simulink model "main_to_linearize"  (R2025b)
settings: Solver=FixedStepAuto  StartTime=0  StopTime=100  FixedStep=sample_time  RelTol=1e-3
undefined symbols (not defined in the file or in its folder): A_cut_in, control_allocator_matrix, f_xy_tf, fractalcoef, G_rate, initial_euler, K_coeff, mav_inertia_ctrl, mav_mass, phase_lag, thrust_coeff_bot, thrust_coeff_top, thrust_tf, top_motor_arm, torque_coeff_bot, torque_coeff_top
libraries: aerolibobsolete x1, matrix_library x1, aerolibutil x1, uavutilslib x1, sensorgpslib x1, mspsensorlib x1, sharedtransform x1
settings Model: Creator=tommy  LastModifiedBy=tommy
settings DataIOCC: SaveFormat=StructureWithTime
settings OptimizationCC: BlockReduction=off  DefaultParameterBehavior=Inlined  UseDivisionForNetSlopeComputation=on  GainParamInheritBuiltInType=on  UseFloatMulNetSlope=on  InlineInvariantSignals=on  OptimizeBlockIOStorage=off  BufferReuse=off  EnhancedBackFolding=on  BooleansAsBitfields=on  PassReuseOutputArgsAs=Individual arguments  StateBitsets=on  DataBitsets=on  ZeroExternalMemoryAtStartup=off  ZeroInternalMemoryAtStartup=off  NoFixptDivByZeroProtection=on  EfficientFloat2IntCast=on  LifeSpan=1  OptimizeBlockOrder=speed  DifferentSizesBufferReuse=on  EfficientTunableParamExpr=on
settings DebuggingCC: AlgebraicLoopMsg=none  ParameterTunabilityLossMsg=error
settings HardwareCC: ProdBitPerPointer=32.0  ProdBitPerSizeT=32.0  ProdBitPerPtrDiffT=32.0  ProdLargestAtomicInteger=Long  ProdLargestAtomicFloat=Double  ProdWordSize=32.0  ProdLongLongMode=on  ProdHWDeviceType=ARM Compatible->ARM Cortex-M
settings SFSimCC: MATLABDynamicMemAlloc=off  SimTargetLang=C++  SimDLTargetLibrary=mkl-dnn
settings RTWCC: SystemTargetFile=ert.tlc  TemplateMakefile=ert_default_tmf  TargetLang=C++  Description=Embedded Coder
settings CodeAppCC: ForceParamTrailComments=on  IgnoreCustomStorageClasses=off  OperatorAnnotations=on  SimulinkDataObjDesc=on  SFDataObjDesc=on  CustomSymbolStrGlobalVar=rt$N$M  CustomSymbolStrType=$N$M  CustomSymbolStrFcn=$N$M$F  CustomSymbolStrMacro=$N$M  InsertBlockDesc=on
settings ERTTargetCC: RootIOFormat=Structure reference  ERTCustomFileTemplate=example_file_process.tlc  ERTFilePackagingFormat=CompactWithDataFile  TargetLangStandard=C++11 (ISO)  GenerateSampleERTMain=on  IncludeMdlTerminateFcn=off  CombineSignalStateStructs=on  SuppressErrorStatus=on  SupportAbsoluteTime=off  CodeInterfacePackaging=C++ class  SupportComplex=off

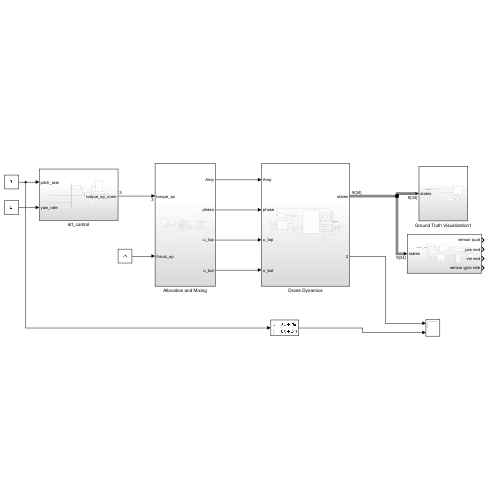
[thumbnail: Simulink's stored preview of the top-level diagram]
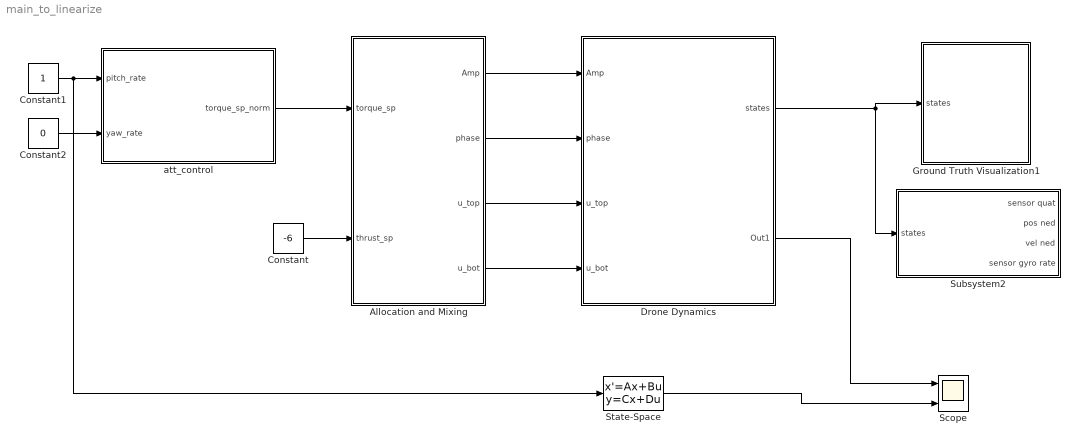
== system main_to_linearize ==
  Allocation and Mixing : Subsystem
  Constant : Constant  Value=-6
  Constant1 : Constant
  Constant2 : Constant  Value=0
  Drone Dynamics : Subsystem
  Ground Truth Visualization1 : Subsystem
  Scope : Scope  NumInputPorts=2
      settings: ActiveDisplayYMinimum=-0.027502183386848192  ActiveDisplayYMaximum=0.021746809856548664  DataLoggingVariableName=ScopeData2
  State-Space : StateSpace  A=G_rate.A  B=G_rate.B  C=G_rate.C  D=G_rate.D  InitialCondition=0
  Subsystem2 : Subsystem
  att_control : Subsystem
  wires:
  Drone Dynamics/1(states) -> Subsystem2/1(states), Ground Truth Visualization1/1(states)
  Allocation and Mixing/2(phase) -> Drone Dynamics/2(phase)
  Allocation and Mixing/3(u_top) -> Drone Dynamics/3(u_top)
  Allocation and Mixing/4(u_bot) -> Drone Dynamics/4(u_bot)
  Allocation and Mixing/1(Amp) -> Drone Dynamics/1(Amp)
  Constant/1 -> Allocation and Mixing/2(thrust_sp)
  att_control/1(torque_sp_norm) -> Allocation and Mixing/1(torque_sp)
  Constant2/1 -> att_control/2(yaw_rate)
  Drone Dynamics/2(Out1) -> Scope/1
  State-Space/1 -> Scope/2
  Constant1/1 -> State-Space/1, att_control/1(pitch_rate)

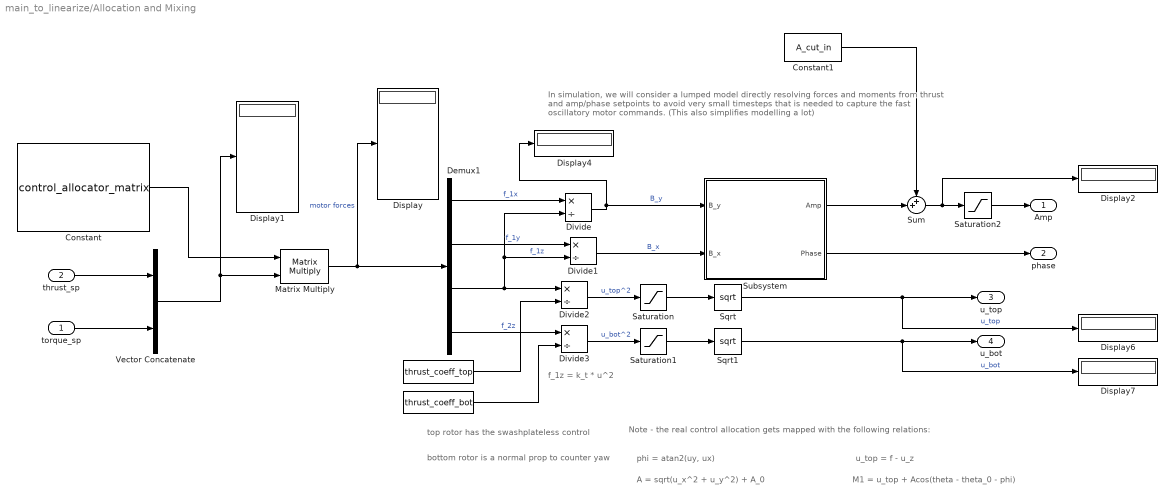
== system main_to_linearize/Allocation and Mixing ==
  note: f_1z = k_t * u^2
  note: u_top = f - u_z
  note: In simulation, we will consider a lumped model directly resolving forces and moments from thrust and amp/phase setpoints to avoid very small timesteps that is needed to capture the fast oscillatory motor commands. (This also simplifies modelling a lot)
  note: phi = atan2(uy, ux)
  note: A = sqrt(u_x^2 + u_y^2) + A_0
  note: top rotor has the swashplateless control
  note: bottom rotor is a normal prop to counter yaw
  note: Note - the real control allocation gets mapped with the following relations:
  note: M1 = u_top + Acos(theta - theta_0 - phi)
  torque_sp : Inport
  thrust_sp : Inport  Port=2
  " " : Constant  Value=thrust_coeff_top
  "  " : Constant  Value=thrust_coeff_bot
  Constant : Constant  Value=control_allocator_matrix
  Constant1 : Constant  Value=A_cut_in
  Demux1 : Demux
  Display{,1..2,4,6..7} (6 alike) : Display
  Divide{,1..3} (4 alike) : Product  Inputs=*/
  Matrix Multiply : Product  Multiplication=Matrix(*)
  Saturation : Saturate  UpperLimit=1  LowerLimit=0
  Saturation1 : Saturate  UpperLimit=1  LowerLimit=0
  Saturation2 : Saturate  UpperLimit=0.3  LowerLimit=0
  Sqrt : Sqrt
  Sqrt1 : Sqrt
  Subsystem : Subsystem
  Sum : Sum  Inputs=++|
  Vector Concatenate : Concatenate
  Amp : Outport
  phase : Outport  Port=2
  u_top : Outport  Port=3
  u_bot : Outport  Port=4
  wires:
  Divide/1 -> Subsystem/1(B_y), Display4/1  "B_y"
  Demux1/2 -> Divide1/1  "f_1y"
  Sqrt/1 -> u_top/1, Display6/1  "u_top"
  Sqrt1/1 -> u_bot/1, Display7/1  "u_bot"
  torque_sp/1 -> Vector Concatenate/2
  Constant/1 -> Matrix Multiply/1
  thrust_sp/1 -> Vector Concatenate/1
  Vector Concatenate/1 -> Display1/1, Matrix Multiply/2
  Matrix Multiply/1 -> Display/1, Demux1/1  "motor forces"
  Sum/1 -> Display2/1, Saturation2/1
  Constant1/1 -> Sum/1
  Saturation2/1 -> Amp/1
  Demux1/1 -> Divide/1  "f_1x"
  Demux1/3 -> Divide/2, Divide1/2, Divide2/1  "f_1z"
  Demux1/4 -> Divide3/1  "f_2z"
  " "/1 -> Divide2/2
  "  "/1 -> Divide3/2
  Divide2/1 -> Saturation/1  "u_top^2"
  Divide3/1 -> Saturation1/1  "u_bot^2"
  Saturation/1 -> Sqrt/1
  Saturation1/1 -> Sqrt1/1
  Divide1/1 -> Subsystem/2(B_x)  "B_x"
  Subsystem/2(Phase) -> phase/1
  Subsystem/1(Amp) -> Sum/2

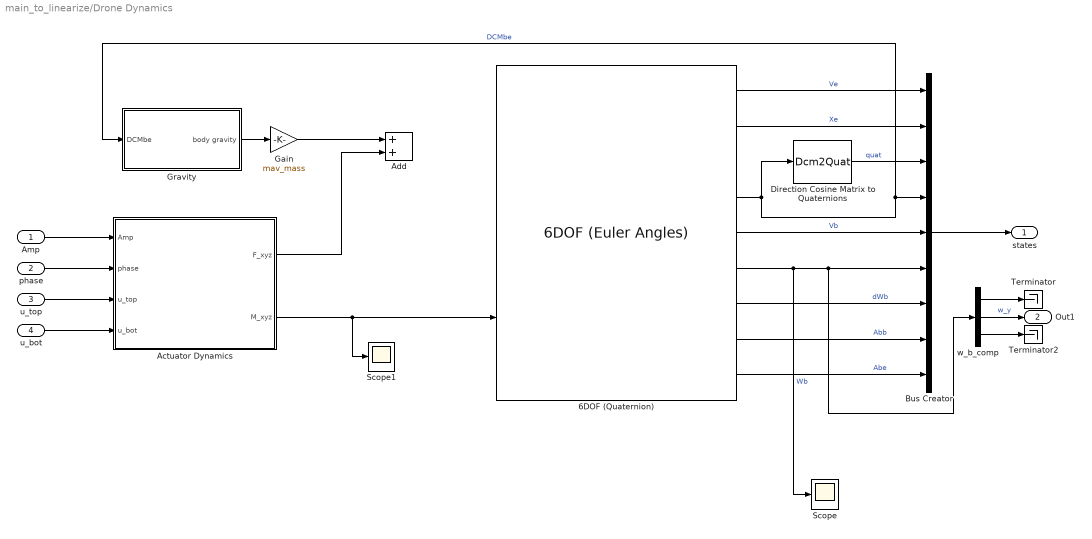
== system main_to_linearize/Drone Dynamics ==
  Amp : Inport
  phase : Inport  Port=2
  u_top : Inport  Port=3
  u_bot : Inport  Port=4
  6DOF (Quaternion) : aerolibobsolete/6DOF (Euler Angles)  units=Metric (MKS)  mtype=Fixed  rep=Quaternion  xme_0=[0 0 0]  Vm_0=[0 0 0]  eul_0=initial_euler  pm_0=[0 0 0]  mass_0=mav_mass  mass_e=0.5  mass_f=2.0  inertia=mav_inertia  inertia_e=eye(3)  inertia_f=2*eye(3)  k_quat=1.0  vre_flag=on  abi_flag=on  aMode=0  xme_statename=''  Vm_statename=''  eul_statename=''  quat_statename=''  pm_statename=''  mass_statename=''
  Actuator Dynamics : Subsystem
  Add : Sum
  Bus Creator : BusCreator  Inputs=9
  Direction Cosine Matrix to Quaternions : Dcm2Quat
  Gain : Gain  Gain=mav_mass
  Gravity : Subsystem
  Scope : Scope
      settings: ActiveDisplayYMinimum=-3.1765505415243829  ActiveDisplayYMaximum=3.0646959132907146  DataLoggingVariableName=ScopeData8
  Scope1 : Scope
      settings: ActiveDisplayYMinimum=-0.093468111798381326  ActiveDisplayYMaximum=0.1127572791811684  DataLoggingVariableName=ScopeData5
  Terminator : Terminator
  Terminator2 : Terminator
  w_b_comp : Demux  Outputs=3
  states : Outport
  Out1 : Outport  Port=2
  wires:
  6DOF (Quaternion)/7 -> Bus Creator/7  "dWb"
  6DOF (Quaternion)/8 -> Bus Creator/8  "Abb"
  6DOF (Quaternion)/6 -> Scope/1, w_b_comp/1, Bus Creator/6  "Wb"
  u_bot/1 -> Actuator Dynamics/4(u_bot)
  Bus Creator/1 -> states/1
  6DOF (Quaternion)/9 -> Bus Creator/9  "Abe"
  phase/1 -> Actuator Dynamics/2(phase)
  6DOF (Quaternion)/1 -> Bus Creator/1  "Ve"
  6DOF (Quaternion)/2 -> Bus Creator/2  "Xe"
  Amp/1 -> Actuator Dynamics/1(Amp)
  6DOF (Quaternion)/5 -> Bus Creator/5  "Vb"
  6DOF (Quaternion)/4 -> Bus Creator/4, Gravity/1(DCMbe), Direction Cosine Matrix to Quaternions/1  "DCMbe"
  Actuator Dynamics/1(F_xyz) -> Add/2
  Gravity/1(body gravity) -> Gain/1
  Gain/1 -> Add/1
  Actuator Dynamics/2(M_xyz) -> Scope1/1, 6DOF (Quaternion)/2
  Direction Cosine Matrix to Quaternions/1 -> Bus Creator/3  "quat"
  u_top/1 -> Actuator Dynamics/3(u_top)
  w_b_comp/1 -> Terminator/1
  w_b_comp/3 -> Terminator2/1
  w_b_comp/2 -> Out1/1  "w_y"

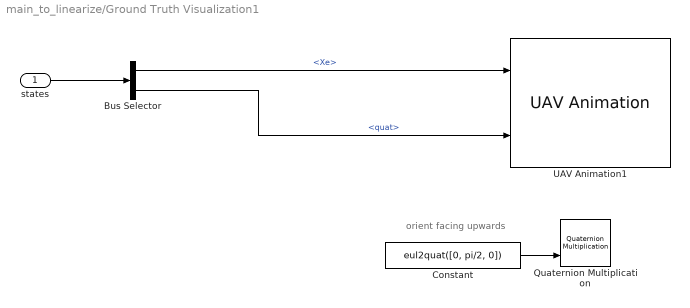
== system main_to_linearize/Ground Truth Visualization1 ==
  note: orient facing upwards
  states : Inport
  Bus Selector : BusSelector  OutputSignals=Xe,quat
  Constant : Constant  Value=eul2quat([0, pi/2, 0])  VectorParams1D=off
  Quaternion Multiplication : aerolibutil/Quaternion Multiplication
  UAV Animation1 : uavutilslib/UAV Animation  NumUAV=1  DynamicUAVConfig=off  UAVType=Multirotor  UAVSize=1  UAVColor=[1 0 0]  UAVTrajectoryAlpha=1  InertialZDirection=Down  RotationFormat=Quaternion  DrawMarkers=off  SampleTime=0.05
  wires:
  states/1 -> Bus Selector/1
  Bus Selector/1 -> UAV Animation1/1  "<Xe>"
  Bus Selector/2 -> UAV Animation1/2  "<quat>"
  Constant/1 -> Quaternion Multiplication/2

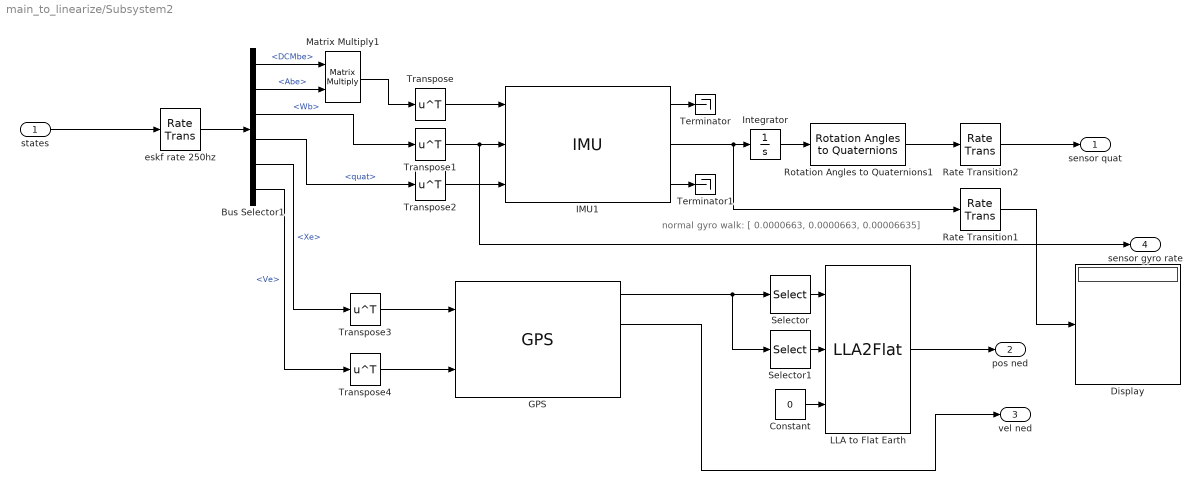
== system main_to_linearize/Subsystem2 ==
  note: normal gyro walk: [ 0.0000663, 0.0000663, 0.00006635]
  states : Inport
  Bus Selector1 : BusSelector  OutputSignals=DCMbe,Abe,Wb,quat,Xe,Ve
  Constant : Constant  Value=0
  Display : Display
  GPS : sensorgpslib/GPS  DispRefFrame=NED  PositionInputFormat=Local  ReferenceLocation=[ 43.660624994362166, -79.39579849130422, 0 ]  HorizontalPositionAccuracy=1.6  VerticalPositionAccuracy=2  VelocityAccuracy=0.1  DecayFactor=0.999  SeedDouble=67  SimulateUsing=Interpreted execution
      settings: LibrarySourceBlock=uavsimlib/GPS
  IMU1 : mspsensorlib/IMU  DispRefFrame=NED  TemperaturePort=off  Temperature=0  MagneticFieldPort=off  MagneticFieldNED=[ 27.5550, -2.4169, -16.0849 ]  MagneticFieldENU=[ -2.4169, 27.5550, 16.0849 ]  SeedDouble=67  SimulateUsing=Interpreted execution  AccelParamsMeasurementRange=Inf  AccelParamsResolution=0  AccelParamsConstantBias=[ 0, 0, 0 ]  AccelParamsAxesMisalignment=[ 1, 0, 0; 0, 1, 0; 0, 0, 1 ]  AccelParamsNoiseDensity=[ 0, 0, 0 ]  AccelParamsBiasInstability=[ 0, 0, 0 ]  AccelParamsBiasInstabilityNumerator=fractalcoef().Numerator  AccelParamsBiasInstabilityDenominator=fractalcoef().Denominator  AccelParamsRandomWalk=[ 0, 0, 0 ]  AccelParamsNoiseType=double-sided  AccelParamsTemperatureBias=[ 0, 0, 0 ]  AccelParamsTemperatureScaleFactor=[ 0, 0, 0 ]  GyroParamsMeasurementRange=Inf  GyroParamsResolution=0  GyroParamsConstantBias=[ 0, 0, 0 ]  GyroParamsAxesMisalignment=[ 100, 0, 0; 0, 100, 0; 0, 0, 100 ]  GyroParamsAccelerationBias=[ 0, 0, 0 ]  GyroParamsNoiseDensity=[0, 0, 0]  GyroParamsBiasInstability=[ 0, 0, 0 ]  GyroParamsBiasInstabilityNumerator=fractalcoef().Numerator  GyroParamsBiasInstabilityDenominator=fractalcoef().Denominator  GyroParamsRandomWalk=[ 0, 0, 0 ]  GyroParamsNoiseType=double-sided  GyroParamsTemperatureBias=[ 0, 0, 0 ]  GyroParamsTemperatureScaleFactor=[ 0, 0, 0 ]  MagParamsMeasurementRange=Inf  MagParamsResolution=0  MagParamsConstantBias=[ 0, 0, 0 ]  MagParamsAxesMisalignment=[ 100, 0, 0; 0, 100, 0; 0, 0, 100 ]  MagParamsNoiseDensity=[ 0, 0, 0 ]  MagParamsBiasInstability=[ 0, 0, 0 ]  MagParamsBiasInstabilityNumerator=fractalcoef().Numerator  MagParamsBiasInstabilityDenominator=fractalcoef().Denominator  MagParamsRandomWalk=[ 0, 0, 0 ]  MagParamsNoiseType=double-sided  MagParamsTemperatureBias=[ 0, 0, 0 ]  MagParamsTemperatureScaleFactor=[ 0, 0, 0 ]
  Integrator : Integrator  InitialCondition=initial_euler
  LLA to Flat Earth : LLA2Flat  LL0=[43.660624994362166, -79.39579849130422]
  Matrix Multiply1 : Product  Multiplication=Matrix(*)
  Rate Transition1 : RateTransition  OutPortSampleTime=1/1000
  Rate Transition2 : RateTransition  OutPortSampleTime=1/250
  Rotation Angles to Quaternions1 : sharedtransform/Rotation Angles to Quaternions  rotationOrder=XYZ  aMode=aMode
  Selector : Selector  InputPortWidth=3  IndexOptions=Index vector (dialog)  Indices=[1 2]  OutputSizes=1
  Selector1 : Selector  InputPortWidth=3  IndexOptions=Index vector (dialog)  Indices=[3]  OutputSizes=1
  Terminator : Terminator
  Terminator1 : Terminator
  Transpose{,1..4} (5 alike) : Math  Operator=transpose
  eskf rate 250hz : RateTransition  OutPortSampleTime=1/250
  sensor quat : Outport
  pos ned : Outport  Port=2
  vel ned : Outport  Port=3
  sensor gyro rate : Outport  Port=4
  wires:
  Transpose1/1 -> IMU1/2, sensor gyro rate/1
  IMU1/2 -> Integrator/1, Rate Transition1/1
  Matrix Multiply1/1 -> Transpose/1
  Transpose/1 -> IMU1/1
  Integrator/1 -> Rotation Angles to Quaternions1/1
  Transpose2/1 -> IMU1/3
  Bus Selector1/4 -> Transpose2/1  "<quat>"
  Bus Selector1/3 -> Transpose1/1  "<Wb>"
  Rotation Angles to Quaternions1/1 -> Rate Transition2/1
  states/1 -> eskf rate 250hz/1
  eskf rate 250hz/1 -> Bus Selector1/1
  IMU1/1 -> Terminator/1
  IMU1/3 -> Terminator1/1
  Bus Selector1/1 -> Matrix Multiply1/1  "<DCMbe>"
  Bus Selector1/2 -> Matrix Multiply1/2  "<Abe>"
  Rate Transition1/1 -> Display/1
  Rate Transition2/1 -> sensor quat/1
  GPS/1 -> Selector1/1, Selector/1
  Selector/1 -> LLA to Flat Earth/1
  Selector1/1 -> LLA to Flat Earth/2
  Constant/1 -> LLA to Flat Earth/3
  GPS/2 -> vel ned/1
  LLA to Flat Earth/1 -> pos ned/1
  Bus Selector1/6 -> Transpose4/1  "<Ve>"
  Bus Selector1/5 -> Transpose3/1  "<Xe>"
  Transpose3/1 -> GPS/1
  Transpose4/1 -> GPS/2

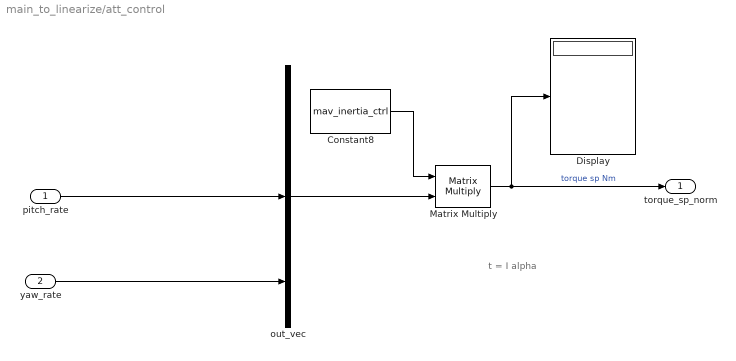
== system main_to_linearize/att_control ==
  note: t = I alpha
  pitch_rate : Inport
  yaw_rate : Inport  Port=2
  Constant8 : Constant  Value=mav_inertia_ctrl
  Display : Display
  Matrix Multiply : Product  Multiplication=Matrix(*)
  out_vec : Concatenate  NumInputs=3
  torque_sp_norm : Outport
  wires:
  Matrix Multiply/1 -> Display/1, torque_sp_norm/1  "torque sp Nm"
  Constant8/1 -> Matrix Multiply/1
  out_vec/1 -> Matrix Multiply/2
  pitch_rate/1 -> out_vec/2
  yaw_rate/1 -> out_vec/3

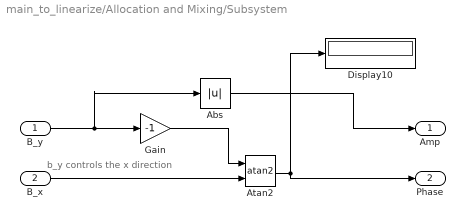
== system main_to_linearize/Allocation and Mixing/Subsystem ==
  note: b_y controls the x direction
  B_y : Inport
  B_x : Inport  Port=2
  Abs : Abs  SaturateOnIntegerOverflow=off
  Atan2 : Trigonometry  Operator=atan2
  Display10 : Display
  Gain : Gain  Gain=-1
  Amp : Outport
  Phase : Outport  Port=2
  wires:
  B_x/1 -> Atan2/2
  B_y/1 -> Abs/1, Gain/1
  Atan2/1 -> Phase/1, Display10/1
  Gain/1 -> Atan2/1
  Abs/1 -> Amp/1

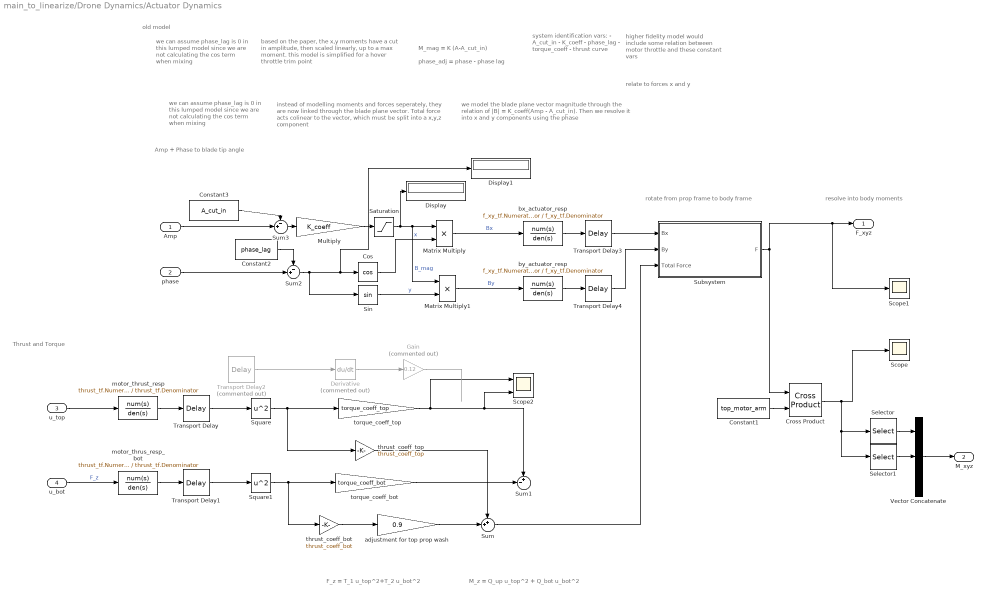
== system main_to_linearize/Drone Dynamics/Actuator Dynamics ==
  note: Amp + Phase to blade tip angle
  note: Thrust and Torque
  note: old model
  note: relate to forces x and y
  note: we can assume phase_lag is 0 in this lumped model since we are not calculating the cos term when mixing
  note: higher fidelity model would include some relation between motor throttle and these constant vars
  note: system identification vars:
      | - A_cut_in
      | - K_coeff
      | - phase_lag
      | - torque_coeff
      | - thrust curve
  note: M_mag = K (A-A_cut_in)
  note: based on the paper, the x,y moments have a cut in amplitude, then scaled linearly, up to a max moment. this model is simplified for a hover throttle trim point
  note: phase_adj = phase - phase lag
  note: M_z = Q_up u_top^2 + Q_bot u_bot^2
  note: F_z = T_1 u_top^2+T_2 u_bot^2
  note: resolve into body moments
  note: we can assume phase_lag is 0 in this lumped model since we are not calculating the cos term when mixing
  note: instead of modelling moments and forces seperately, they are now linked through the blade plane vector. Total force acts colinear to the vector, which must be split into a x,y,z component
  note: we model the blade plane vector magnitude through the relation of |B| = K_coeff(Amp - A_cut_in). Then we resolve it into x and y components using the phase
  note: rotate from prop frame to body frame
  Amp : Inport
  phase : Inport  Port=2
  u_top : Inport  Port=3
  u_bot : Inport  Port=4
  Constant1 : Constant  Value=top_motor_arm
  Constant2 : Constant  Value=phase_lag
  Constant3 : Constant  Value=A_cut_in
  Cos : Trigonometry  Operator=cos
  Cross Product : matrix_library/Cross Product
  Derivative : Derivative  Commented=on
  Display : Display
  Display1 : Display
  Gain : Gain  Commented=on  Gain=0.12
  Matrix Multiply : Product
  Matrix Multiply1 : Product
  Multiply : Gain  Gain=K_coeff
  Saturation : Saturate  UpperLimit=inf  LowerLimit=0
  Scope : Scope
      settings: ActiveDisplayYMinimum=-0.0046517365862840283  ActiveDisplayYMaximum=0.012758813227963812
  Scope1 : Scope
      settings: ActiveDisplayYMinimum=-1  ActiveDisplayYMaximum=1
  Scope2 : Scope  NumInputPorts=2
      settings: ActiveDisplayYMinimum=-0.016923057380667912  ActiveDisplayYMaximum=0.1375268910048818  DataLoggingVariableName=ScopeData10
  Selector : Selector  InputPortWidth=3  IndexOptions=Index vector (dialog)  Indices=[1]  OutputSizes=1
  Selector1 : Selector  InputPortWidth=3  IndexOptions=Index vector (dialog)  Indices=[2]  OutputSizes=1
  Sin : Trigonometry
  Square : Math  Operator=square
  Square1 : Math  Operator=square
  Subsystem : Subsystem
  Sum : Sum  Inputs=++|
  Sum1 : Sum  Inputs=+-|
  Sum2 : Sum  Inputs=-+|
  Sum3 : Sum  Inputs=-+|
  Transport Delay : TransportDelay  DelayTime=0.15  TransDelayFeedthrough=on  PadeOrder=1
  Transport Delay1 : TransportDelay  DelayTime=0.15  TransDelayFeedthrough=on  PadeOrder=1
  Transport Delay2 : TransportDelay  Commented=on  DelayTime=0.1
  Transport Delay3 : TransportDelay  DelayTime=0.1  TransDelayFeedthrough=on  PadeOrder=1
  Transport Delay4 : TransportDelay  DelayTime=0.1  TransDelayFeedthrough=on  PadeOrder=1
  Vector Concatenate : Concatenate  NumInputs=3
  adjustment for top prop wash : Gain  Gain=0.9
  bx_actuator_resp : TransferFcn  Numerator=f_xy_tf.Numerator  Denominator=f_xy_tf.Denominator
  by_actuator_resp : TransferFcn  Numerator=f_xy_tf.Numerator  Denominator=f_xy_tf.Denominator
  motor_thrus_resp_bot : TransferFcn  Numerator=thrust_tf.Numerator  Denominator=thrust_tf.Denominator
  motor_thrust_resp : TransferFcn  Numerator=thrust_tf.Numerator  Denominator=thrust_tf.Denominator
  thrust_coeff_bot : Gain  Gain=thrust_coeff_bot
  thrust_coeff_top : Gain  Gain=thrust_coeff_top
  torque_coeff_bot : Gain  Gain=torque_coeff_bot
  torque_coeff_top : Gain  Gain=torque_coeff_top
  F_xyz : Outport
  M_xyz : Outport  Port=2
  wires:
  u_bot/1 -> motor_thrus_resp_bot/1  "F_z"
  Constant2/1 -> Sum2/1
  phase/1 -> Sum2/2
  Sum2/1 -> Sin/1, Cos/1, Display1/1
  Amp/1 -> Sum3/2
  Constant3/1 -> Sum3/1
  Sum3/1 -> Multiply/1
  Multiply/1 -> Saturation/1
  Cos/1 -> Matrix Multiply/2  "x"
  Matrix Multiply1/1 -> by_actuator_resp/1  "By"
  Sin/1 -> Matrix Multiply1/2  "y"
  Saturation/1 -> Display/1, Matrix Multiply1/1, Matrix Multiply/1  "B_mag"
  Constant1/1 -> Cross Product/2
  Cross Product/1 -> Selector1/1, Selector/1, Scope/1
  Subsystem/1(F) -> Scope1/1, F_xyz/1, Cross Product/1
  by_actuator_resp/1 -> Transport Delay4/1
  bx_actuator_resp/1 -> Transport Delay3/1
  Square/1 -> torque_coeff_top/1, thrust_coeff_top/1
  Square1/1 -> thrust_coeff_bot/1, torque_coeff_bot/1
  Vector Concatenate/1 -> M_xyz/1
  Selector/1 -> Vector Concatenate/1
  Selector1/1 -> Vector Concatenate/2
  torque_coeff_bot/1 -> Sum1/2
  Matrix Multiply/1 -> bx_actuator_resp/1  "Bx"
  thrust_coeff_bot/1 -> adjustment for top prop wash/1
  torque_coeff_top/1 -> Scope2/2, Sum1/1, Scope2/1
  u_top/1 -> motor_thrust_resp/1
  thrust_coeff_top/1 -> Sum/1
  adjustment for top prop wash/1 -> Sum/2
  Derivative/1 -> Gain/1
  Gain/1 -> ?
  Transport Delay2/1 -> Derivative/1
  Sum/1 -> Subsystem/3(Total Force)
  ? -> Transport Delay2/1
  motor_thrus_resp_bot/1 -> Transport Delay1/1
  motor_thrust_resp/1 -> Transport Delay/1
  Transport Delay/1 -> Square/1
  Transport Delay1/1 -> Square1/1
  Transport Delay3/1 -> Subsystem/1(Bx)
  Transport Delay4/1 -> Subsystem/2(By)

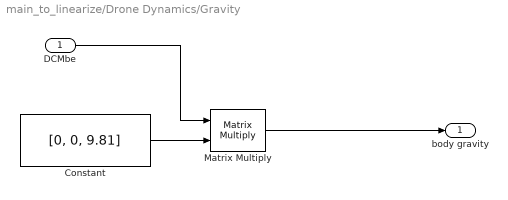
== system main_to_linearize/Drone Dynamics/Gravity ==
  DCMbe : Inport
  Constant : Constant  Value=[0, 0, 9.81]
  Matrix Multiply : Product  Multiplication=Matrix(*)
  body gravity : Outport
  wires:
  DCMbe/1 -> Matrix Multiply/1
  Constant/1 -> Matrix Multiply/2
  Matrix Multiply/1 -> body gravity/1

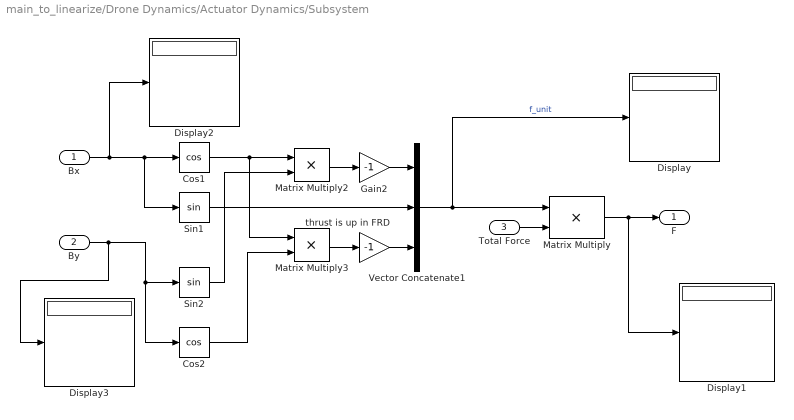
== system main_to_linearize/Drone Dynamics/Actuator Dynamics/Subsystem ==
  Bx : Inport
  By : Inport  Port=2
  Total Force : Inport  Port=3
  Cos1 : Trigonometry  Operator=cos
  Cos2 : Trigonometry  Operator=cos
  Display{,1..3} (4 alike) : Display
  Gain2 : Gain  Gain=-1
  Matrix Multiply : Product
  Matrix Multiply2 : Product
  Matrix Multiply3 : Product
  Sin1 : Trigonometry
  Sin2 : Trigonometry
  Vector Concatenate1 : Concatenate  NumInputs=3
  thrust is up in FRD : Gain  Gain=-1
  F : Outport
  wires:
  Sin1/1 -> Vector Concatenate1/2
  Bx/1 -> Display2/1, Sin1/1, Cos1/1
  Cos1/1 -> Matrix Multiply3/1, Matrix Multiply2/1
  Cos2/1 -> Matrix Multiply3/2
  By/1 -> Display3/1, Cos2/1, Sin2/1
  Sin2/1 -> Matrix Multiply2/2
  Vector Concatenate1/1 -> Display/1, Matrix Multiply/1  "f_unit"
  Total Force/1 -> Matrix Multiply/2
  Matrix Multiply/1 -> Display1/1, F/1
  Matrix Multiply2/1 -> Gain2/1
  Matrix Multiply3/1 -> thrust is up in FRD/1
  Gain2/1 -> Vector Concatenate1/1
  thrust is up in FRD/1 -> Vector Concatenate1/3
